simulink model "simulation"  (R2019b)
settings: Solver=VariableStepAuto  StartTime=0.0  StopTime=10.0  RelTol=1e-3
values from neighbouring files (symbols this model uses):
  Abar = [Ap zeros(np,m); Cp zeros(m,m)]    [main.m]
  B = [Bp; zeros(m,m)]    [main.m]
  Bc = [zeros(np,m); -eye(m)]    [main.m]
  Kbl = -K    [main.m]
  Lambda = eye(m)    [main.m]
settings Model: Creator=aleix  LastModifiedBy=aleix

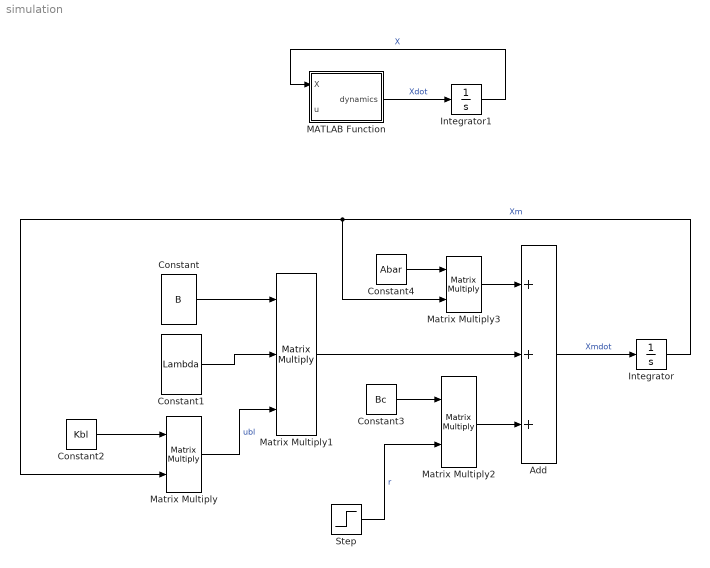
== system simulation ==
  Add : Sum  Inputs=3
  Constant : Constant  Value=B
  Constant1 : Constant  Value=Lambda
  Constant2 : Constant  Value=Kbl
  Constant3 : Constant  Value=Bc
  Constant4 : Constant  Value=Abar
  Integrator : Integrator
  Integrator1 : Integrator
  MATLAB Function : MATLAB Function  TreatAsAtomicUnit=on
  Matrix Multiply : Product  Multiplication=Matrix(*)
  Matrix Multiply1 : Product  Inputs=3  Multiplication=Matrix(*)
  Matrix Multiply2 : Product  Multiplication=Matrix(*)
  Matrix Multiply3 : Product  Multiplication=Matrix(*)
  Step : Step  SampleTime=0
  wires:
  Add/1 -> Integrator/1  "Xmdot"
  Integrator/1 -> Matrix Multiply3/2, Matrix Multiply/2  "Xm"
  Matrix Multiply3/1 -> Add/1
  Matrix Multiply1/1 -> Add/2
  Constant2/1 -> Matrix Multiply/1
  Matrix Multiply/1 -> Matrix Multiply1/3  "ubl"
  Constant/1 -> Matrix Multiply1/1
  Constant1/1 -> Matrix Multiply1/2
  Matrix Multiply2/1 -> Add/3
  Constant3/1 -> Matrix Multiply2/1
  Step/1 -> Matrix Multiply2/2  "r"
  Constant4/1 -> Matrix Multiply3/1
  MATLAB Function/1(dynamics) -> Integrator1/1  "Xdot"
  Integrator1/1 -> MATLAB Function/1(X)  "X"

== matlab function simulation/MATLAB Function ==
  data: X input; dynamics output; u input
function dynamics = fcn(X,u)

% Dynamics
%pos                    = X(1:3);
phi                    = X(4);
theta                  = X(5);
psi                    = X(6);
vel_x                  = X(7);
vel_y                  = X(8);
vel_z                  = X(9);
p                      = X(10);
q                      = X(11);
r                      = X(12);
deltaU1                = u(1);
U2                     = u(2);
U3                     = u(3);
U4                     = u(4);
sphi   = sin(phi);
stheta = sin(theta);
spsi   = sin(psi);
cphi   = cos(phi);
ctheta = cos(theta);
cpsi   = cos(psi);
ttheta = tan(theta);

pos_dot_x     = vel_x;
pos_dot_y     = vel_y;
pos_dot_z     = vel_z;
orient_dot_x  = p + r.*(cphi.*ttheta) + q.*(sphi.*ttheta);
orient_dot_y  = q.*cphi - r.*sphi;
orient_dot_z  = r.*cphi./ctheta + q.*sphi./ctheta;
vel_dot_x     = deltaU1.*(sphi.*spsi + cphi.*cpsi.*stheta)./m - Axyz(1).*vel_x./m;
vel_dot_y     = deltaU1.*(cphi.*spsi.*stheta - cpsi.*sphi)./m - Axyz(2).*vel_y./m;
vel_dot_z     = deltaU1.*(cphi.*ctheta)./m - g                - Axyz(3).*vel_z./m;
rate_dot_x    = ((Iy - Iz).*r.*q + U2)./Ix;
rate_dot_y    = ((Iz - Ix).*p.*r + U3)./Iy;
rate_dot_z    = ((Ix - Iy).*p.*q + U4)./Iz;

output_dynamics   = [pos_dot_x, pos_dot_y, pos_dot_z, ...
    orient_dot_x, orient_dot_y, orient_dot_z, vel_dot_x, vel_dot_y, vel_dot_z,  ...
    rate_dot_x, rate_dot_y, rate_dot_z, eyI...];

% g      = input.auxdata.g;
% m      = input.auxdata.M;
% Ix     = input.auxdata.Ix;
% Iy     = input.auxdata.Iy;
% Iz     = input.auxdata.Iz;
